simulink library "Force_Moment_Sublibrary"  (R2019a)
settings: Solver=VariableStepAuto  StartTime=0.0  StopTime=10.0  RelTol=1e-3
undefined symbols (not defined in the file): ENV, Motor, VEH
libraries: simulink x6, Rail_UL x1
settings Model: Creator=John Jr  LastModifiedBy=John Jr

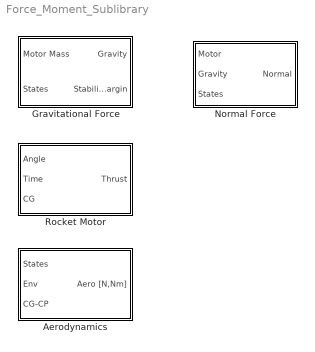
== system Force_Moment_Sublibrary ==
  Aerodynamics : Subsystem  mask{C_d=VEH.C_d, A_ref=VEH.A_ref, C_s=VEH.C_s, A_side=VEH.A_side, z_r=0}
      mask prompts: C_d "Drag Coefficient"; A_ref "Reference area [m^2]"; C_s "Side force coefficient"; A_side "Reference area [m^2]"; z_r "Rail length [m]"
      mask DialogControl DescGroupVar Prompt: Aerodynamics Library
      mask DialogControl DescTextVar Prompt: This block models the aerodynamic forces and moments acting on the vehicle in "body-fixed" coordinates.
      mask DialogControl Control2 Prompt: Drag Force Parameters:
      mask DialogControl Control3 Prompt: Side Force Parameters:
      mask Display:
      | patch([0 1 1 0], [0 0 1 1],[.8 1 1])
      | 
      | port_label('input',1,'\fontname{Cambria Math}States','texmode','on')
      | port_label('input',2,'\fontname{Cambria Math}Env','texmode','on')
      | port_label('input',3,'\fontname{Cambria Math}CP-CG [m]','texmode','on')
      | 
      | port_label('output',1,'\fontname{Cambria Math}Aerodynamics','texmode','on')
  Gravitational Force : Subsystem  mask{g=ENV.g, m=VEH.m, CG1=VEH.CG_1, CG2=VEH.CG_2, CP=VEH.CP, t_b=Motor.t_b}
      mask prompts: g "Gravitational acceleration [m/s^2]"; m "Vehicle mass without motor [kg]"; CG1 "CG on launchpad [m]"; CG2 "CG after motor burn [m]"; CP "Center of pressure [m]"; t_b "Total motor burn time [s]"
      mask DialogControl DescGroupVar Prompt: Gravitational Force Library
      mask DialogControl DescTextVar Prompt: This block models the gravitational force acting on the vehicle, as well as the stability margin as the motor burns.
      mask DialogControl Control2 Prompt: Stability Properties (measured from nosecone):
      mask Display:
      | patch([0 1 1 0], [0 0 1 1],[.8 1 1])
      | 
      | port_label('input',1,'\fontname{Cambria Math}M_{motor} [kg]','texmode','on')
      | port_label('input',2,'\fontname{Cambria Math}States','texmode','on')
      | 
      | port_label('output',1,'\fontname{Cambria Math}Gravity [N]','texmode','on')
      | port_label('output',2,'\fontname{Cambria Math}CG-CP [m]','texmode','on')
  Normal Force : Subsystem
      mask Display:
      | patch([0 1 1 0], [0 0 1 1],[.8 1 1])
      | 
      | port_label('input',1,'\fontname{Cambria Math}Motor','texmode','on')
      | port_label('input',2,'\fontname{Cambria Math}Gravity','texmode','on')
      | port_label('input',3,'\fontname{Cambria Math}States','texmode','on')
      | 
      | port_label('output',1,'\fontname{Cambria Math}Normal [N]','texmode','on')
  Rocket Motor : Subsystem  mask{F_th=Motor.F_th, t_vec=Motor.T_b, t_b=Motor.t_b, m_m=Motor.m_m, m_f=Motor.m_f, k=Motor.k_m, L=VEH.L}
      mask prompts: F_th "Thrust curve force vector"; t_vec "Thrust curve time vector"; t_b "Total motor burn time [s]"; m_m "Empty motor mass [kg]"; m_f "Propellant mass [kg]"; k "Motor variance"; L "Vehicle length [m]"
      mask DialogControl DescGroupVar Prompt: Rocket Motor Library
      mask DialogControl DescTextVar Prompt: This block models the motor's thrust acting on the vehicle, including rotational effects.
      mask Display:
      | patch([0 1 1 0], [0 0 1 1],[.8 1 1])
      | 
      | port_label('input',1,'\fontname{Cambria Math}Angle [rad]','texmode','on')
      | port_label('input',2,'\fontname{Cambria Math}Time [s]','texmode','on')
      | port_label('input',3,'\fontname{Cambria Math}CG [m]','texmode','on')
      | 
      | port_label('output',1,'\fontname{Cambria Math}Motor_{out}','texmode','on')

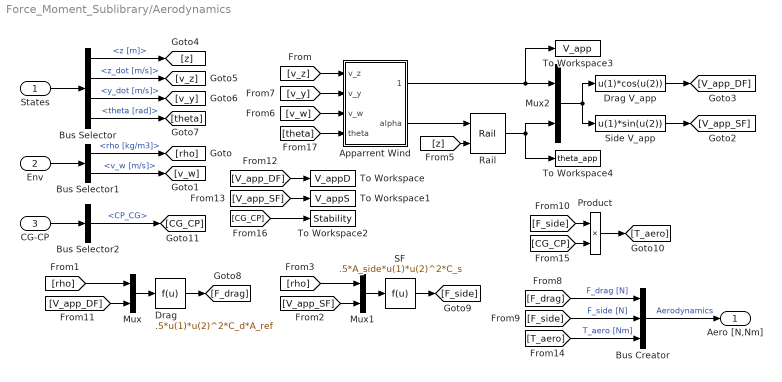
== system Force_Moment_Sublibrary/Aerodynamics ==
  States : Inport
  Env : Inport  Port=2
  CG-CP : Inport  Port=3
  Apparrent Wind : MATLAB Function  TreatAsAtomicUnit=on
  Bus Creator : BusCreator  Inputs=3
  Bus Selector : BusSelector  OutputSignals=Z_g.z [m],Z_g.z_dot [m/s],Y_g.y_dot [m/s],theta.theta [rad]
  Bus Selector1 : BusSelector  OutputSignals=rho [kg/m3],v_w [m/s]
  Bus Selector2 : BusSelector  OutputSignals=CP_CG
  Drag : Fcn  Expr=.5*u(1)*u(2)^2*C_d*A_ref
  Drag V_app : Fcn  Expr=u(1)*cos(u(2))
  Mux : Mux  Inputs=2
  Mux1 : Mux  Inputs=2
  Mux2 : Mux  Inputs=2
  Product : Product
  Rail : Rail_UL/Rail  z_r=ENV.z_r  a_out=0
  SF : Fcn  Expr=.5*A_side*u(1)*u(2)^2*C_s
  Side V_app : Fcn  Expr=u(1)*sin(u(2))
  To Workspace : ToWorkspace  VariableName=V_appD  SampleTime=-1
  To Workspace1 : ToWorkspace  VariableName=V_appS  SampleTime=-1
  To Workspace2 : ToWorkspace  VariableName=Stability  SampleTime=-1
  To Workspace3 : ToWorkspace  VariableName=V_app  SampleTime=-1
  To Workspace4 : ToWorkspace  VariableName=theta_app  SampleTime=-1
  Aero [N,Nm] : Outport
  wires:
  States/1 -> Bus Selector/1
  Bus Selector/1 -> [z]  "<z [m]>"
  Bus Selector/2 -> [v_z]  "<z_dot [m/s]>"
  Bus Selector/3 -> [v_y]  "<y_dot [m/s]>"
  Bus Selector/4 -> [theta]  "<theta [rad]>"
  Env/1 -> Bus Selector1/1
  Bus Selector1/1 -> [rho]  "<rho [kg/m3]>"
  Bus Selector1/2 -> [v_w]  "<v_w [m/s]>"
  Bus Creator/1 -> Aero [N,Nm]/1  "Aerodynamics"
  [F_side] -> Bus Creator/2  "F_side [N]"
  [F_drag] -> Bus Creator/1  "F_drag [N]"
  [F_side] -> Product/1
  Product/1 -> [T_aero]
  [T_aero] -> Bus Creator/3  "T_aero [Nm]"
  [V_app_DF] -> To Workspace/1
  [V_app_SF] -> To Workspace1/1
  CG-CP/1 -> Bus Selector2/1
  [CG_CP] -> Product/2
  [CG_CP] -> To Workspace2/1
  [v_y] -> Apparrent Wind/2(v_y)
  Apparrent Wind/1(v_app) -> To Workspace3/1, Mux2/1
  [theta] -> Apparrent Wind/4(theta)
  Apparrent Wind/2(alpha) -> Rail/1
  [v_z] -> Apparrent Wind/1(v_z)
  Drag V_app/1 -> [V_app_DF]
  [z] -> Rail/2
  Mux2/1 -> Side V_app/1, Drag V_app/1
  Side V_app/1 -> [V_app_SF]
  [v_w] -> Apparrent Wind/3(v_w)
  Rail/1 -> Mux2/2, To Workspace4/1
  [V_app_SF] -> Mux1/2
  [rho] -> Mux1/1
  Mux/1 -> Drag/1
  [rho] -> Mux/1
  Mux1/1 -> SF/1
  SF/1 -> [F_side]
  [V_app_DF] -> Mux/2
  Drag/1 -> [F_drag]
  Bus Selector2/1 -> [CG_CP]  "<CP_CG>"

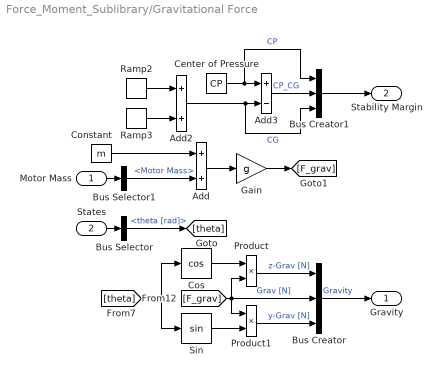
== system Force_Moment_Sublibrary/Gravitational Force ==
  Motor Mass : Inport
  States : Inport  Port=2
  Add : Sum
  Add2 : Sum
  Add3 : Sum  Inputs=+-
  Bus Creator : BusCreator  Inputs=3
  Bus Creator1 : BusCreator  Inputs=3
  Bus Selector : BusSelector  OutputSignals=theta.theta [rad]
  Bus Selector1 : BusSelector  OutputSignals=Motor Mass
  Center of Pressure : Constant  Value=CP
  Constant : Constant  Value=m
  Cos : Trigonometry  Operator=cos
  Gain : Gain  Gain=g
  Product : Product
  Product1 : Product
  Ramp2 : simulink/Sources/Ramp  slope=-(CG1-CG2)/t_b  start=0  InitialOutput=CG1
  Ramp3 : simulink/Sources/Ramp  slope=(CG1-CG2)/t_b  start=t_b  InitialOutput=0
  Sin : Trigonometry
  Gravity : Outport
  Stability Margin : Outport  Port=2
  wires:
  Bus Selector/1 -> [theta]  "<theta [rad]>"
  Bus Selector1/1 -> Add/2  "<Motor Mass>"
  Motor Mass/1 -> Bus Selector1/1
  States/1 -> Bus Selector/1
  Add/1 -> Gain/1
  Constant/1 -> Add/1
  Ramp3/1 -> Add2/2
  Ramp2/1 -> Add2/1
  Center of Pressure/1 -> Bus Creator1/1, Add3/1  "CP"
  Add2/1 -> Bus Creator1/3, Add3/2  "CG"
  [F_grav] -> Bus Creator/2, Product1/1, Product/2  "Grav [N]"
  Gain/1 -> [F_grav]
  Cos/1 -> Product/1
  Sin/1 -> Product1/2
  [theta] -> Sin/1, Cos/1
  Product1/1 -> Bus Creator/3  "y-Grav [N]"
  Product/1 -> Bus Creator/1  "z-Grav [N]"
  Bus Creator/1 -> Gravity/1  "Gravity"
  Bus Creator1/1 -> Stability Margin/1
  Add3/1 -> Bus Creator1/2  "CP_CG"

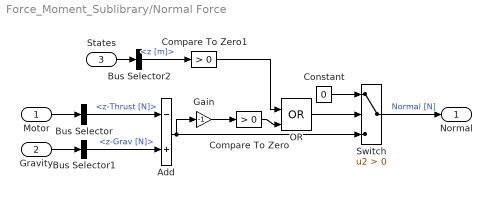
== system Force_Moment_Sublibrary/Normal Force ==
  Motor : Inport
  Gravity : Inport  Port=2
  States : Inport  Port=3
  Add : Sum  Inputs=-+
  Bus Selector : BusSelector  OutputSignals=z-Thrust [N]
  Bus Selector1 : BusSelector  OutputSignals=z-Grav [N]
  Bus Selector2 : BusSelector  OutputSignals=Z_g.z [m]
  Compare To Zero : simulink/Logic and Bit Operations/Compare To Zero  relop=>  OutDataTypeStr=boolean
  Compare To Zero1 : simulink/Logic and Bit Operations/Compare To Zero  relop=>  OutDataTypeStr=boolean
  Constant : Constant  Value=0
  Gain : Gain  Gain=-1
  OR : Logic  Operator=OR  IconShape=distinctive  AllPortsSameDT=off  OutDataTypeStr=boolean
  Switch : Switch  Criteria=u2 > Threshold
  Normal : Outport
  wires:
  States/1 -> Bus Selector2/1
  Motor/1 -> Bus Selector/1
  Gravity/1 -> Bus Selector1/1
  Bus Selector/1 -> Add/1  "<z-Thrust [N]>"
  Bus Selector1/1 -> Add/2  "<z-Grav [N]>"
  Switch/1 -> Normal/1  "Normal [N]"
  Constant/1 -> Switch/1
  Add/1 -> Switch/3, Gain/1
  Bus Selector2/1 -> Compare To Zero1/1  "<z [m]>"
  OR/1 -> Switch/2
  Gain/1 -> Compare To Zero/1
  Compare To Zero/1 -> OR/2
  Compare To Zero1/1 -> OR/1

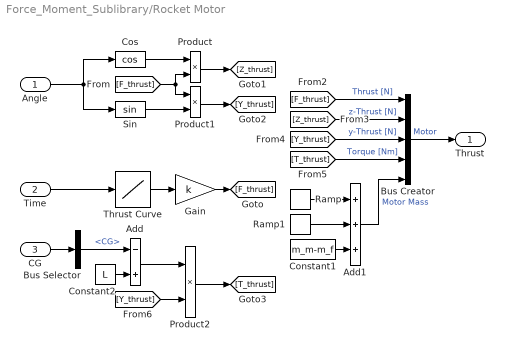
== system Force_Moment_Sublibrary/Rocket Motor ==
  Angle : Inport
  Time : Inport  Port=2
  CG : Inport  Port=3
  Add : Sum  Inputs=-+
  Add1 : Sum  Inputs=+++
  Bus Creator : BusCreator  Inputs=5
  Bus Selector : BusSelector  OutputSignals=CG
  Constant1 : Constant  Value=m_m-m_f
  Constant2 : Constant  Value=L
  Cos : Trigonometry  Operator=cos
  Gain : Gain  Gain=k
  Product : Product
  Product1 : Product
  Product2 : Product
  Ramp : simulink/Sources/Ramp  slope=-m_f/t_b  start=0  InitialOutput=m_f
  Ramp1 : simulink/Sources/Ramp  slope=m_f/t_b  start=t_b  InitialOutput=0
  Sin : Trigonometry
  Thrust Curve : Lookup_n-D  NumberOfTableDimensions=1  BreakpointsForDimension1=t_vec  Table=F_th  InternalRulePriority=Speed  RndMeth=Simplest  InputSameDT=on
  Thrust : Outport
  wires:
  Add1/1 -> Bus Creator/5  "Motor Mass"
  Ramp1/1 -> Add1/2
  Constant1/1 -> Add1/3
  Ramp/1 -> Add1/1
  [T_thrust] -> Bus Creator/4  "Torque [Nm]"
  [Y_thrust] -> Bus Creator/3  "y-Thrust [N]"
  [Z_thrust] -> Bus Creator/2  "z-Thrust [N]"
  [F_thrust] -> Bus Creator/1  "Thrust [N]"
  Bus Creator/1 -> Thrust/1  "Motor"
  Product1/1 -> [Y_thrust]
  Product/1 -> [Z_thrust]
  Sin/1 -> Product1/2
  [F_thrust] -> Product/2, Product1/1
  Cos/1 -> Product/1
  Angle/1 -> Cos/1, Sin/1
  Gain/1 -> [F_thrust]
  Time/1 -> Thrust Curve/1
  Thrust Curve/1 -> Gain/1
  CG/1 -> Bus Selector/1
  Constant2/1 -> Add/2
  Bus Selector/1 -> Add/1  "<CG>"
  Add/1 -> Product2/1
  [Y_thrust] -> Product2/2
  Product2/1 -> [T_thrust]

== matlab function Force_Moment_Sublibrary/Aerodynamics/Apparrent Wind ==
  data: v_z input; v_y input; v_w input; v_app output size=1; alpha output size=1; theta input
function [v_app,alpha] = fcn(v_z,v_y,v_w,theta)

V = [v_y v_z];
V_w = [v_w 0];
V_app = V_w-V;

[theta_V,d_V] = getVangle(V);
if norm(V) == 0
    theta_a = pi/2;
else
    theta_a = acos((-norm(V_w)^2+norm(V)^2+norm(V_app)^2)/(2*norm(V)*norm(V_app)));
end
if V_app(2) > 0
    theta_0 = theta_a-(theta_V*d_V);
else
    theta_0 = theta_a+theta_V*d_V;
end
if V_app(1) >= 0 && V_app(2) <= 0
    alpha = theta_0-theta;
elseif V_app(1) < 0 && V_app(2) <= 0
    alpha = theta_0-theta;
elseif V_app(1) < 0 && V_app(2) > 0
    alpha = -theta_0-theta;
% elseif V_app(1) >= 0 && V_app(2) > 0
else
    alpha = -theta_0-theta;
end
if alpha < -pi
    alpha = 2*pi+alpha;
end
v_app = norm(V_app);
